simulink model "example_simulink_model_wrapper_firmware"  (R2020b)
settings: Solver=ode2  StartTime=0.0  StopTime=inf  FixedStep=0.01  RelTol=1e-3
undefined symbols (not defined in the file or in its folder): constants
settings Model: Creator=ac112430  LastModifiedBy=ac134326
settings DataIOCC: ReturnWorkspaceOutputs=off
settings OptimizationCC: DefaultParameterBehavior=Inlined  DefaultUnderspecifiedDataType=single  PassReuseOutputArgsAs=Individual arguments  EfficientTunableParamExpr=on
settings DebuggingCC: ParameterPrecisionLossMsg=none  ParameterTunabilityLossMsg=error  ArithmeticOperatorsInVariantConditions=warning
settings HardwareCC: ProdBitPerPointer=32  ProdBitPerSizeT=32  ProdBitPerPtrDiffT=32  ProdLargestAtomicInteger=Long  ProdLargestAtomicFloat=Double  ProdIntDivRoundTo=Undefined  ProdWordSize=32  ProdHWDeviceType=ARM Compatible->ARM Cortex
settings ModelReferenceCC: ModelReferenceNumInstancesAllowed=Single  PropagateSignalLabelsOutOfModel=off
settings SFSimCC: SimUseLocalCustomCode=off  MATLABDynamicMemAlloc=off  CustomCodeUndefinedFunction=UseInterfaceOnly
settings RTWCC: Description=Embedded Coder  SystemTargetFile=ert.tlc  GenCodeOnly=on  TemplateMakefile=ert_default_tmf  RTWUseLocalCustomCode=off  IncludeHyperlinkInReport=on
settings CodeAppCC: IgnoreCustomStorageClasses=off  MaxIdLength=63  StateflowObjectComments=on
settings ERTTargetCC: TargetLangStandard=C99 (ISO)  GenerateSampleERTMain=on  SupportNonFinite=off  SupportComplex=off  InlinedParameterPlacement=NonHierarchical  ERTCustomFileTemplate=example_file_process.tlc  ConvertIfToSwitch=off  SuppressUnreachableDefaultCases=off

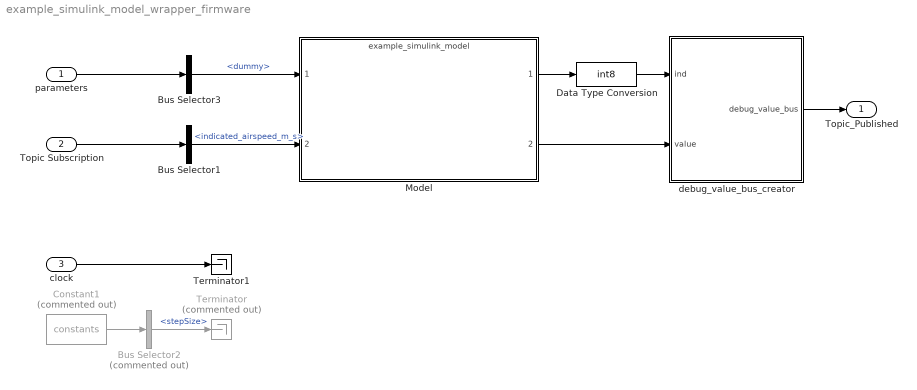
== system example_simulink_model_wrapper_firmware ==
  parameters : Inport  OutDataTypeStr=Bus: parameterBus
  Topic Subscription : Inport  Port=2  OutDataTypeStr=Bus: airspeed_bus
  clock : Inport  Port=3  OutDataTypeStr=single
  Bus Selector1 : BusSelector  OutputSignals=indicated_airspeed_m_s
  Bus Selector2 : BusSelector  Commented=on  OutputSignals=stepSize
  Bus Selector3 : BusSelector  OutputSignals=dummy
  Constant1 : Constant  Commented=on  Value=constants  OutDataTypeStr=Bus: constantsBus
  Data Type Conversion : DataTypeConversion  OutDataTypeStr=int8
  Model : ModelReference  ModelNameDialog=example_simulink_model.slx  SimulationMode=Normal  ModelReferenceVersion=4.3
  Terminator : Terminator  Commented=on
  Terminator1 : Terminator
  debug_value_bus_creator : Subsystem
  Topic_Published : Outport  OutDataTypeStr=Bus: debug_value_bus  SampleTime=[0.01,0]  VectorParamsAs1DForOutWhenUnconnected=off
  wires:
  clock/1 -> Terminator1/1
  parameters/1 -> Bus Selector3/1
  Constant1/1 -> Bus Selector2/1
  Bus Selector2/1 -> Terminator/1  "<stepSize>"
  Topic Subscription/1 -> Bus Selector1/1
  debug_value_bus_creator/1(debug_value_bus) -> Topic_Published/1
  Bus Selector3/1 -> Model/1  "<dummy>"
  Bus Selector1/1 -> Model/2  "<indicated_airspeed_m_s>"
  Model/1 -> Data Type Conversion/1
  Model/2 -> debug_value_bus_creator/2(value)
  Data Type Conversion/1 -> debug_value_bus_creator/1(ind)

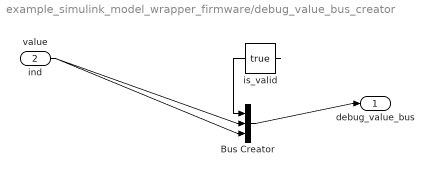
== system example_simulink_model_wrapper_firmware/debug_value_bus_creator ==
  ind : Inport  OutDataTypeStr=int8  PortDimensions=1
  value : Inport  Port=2  OutDataTypeStr=single  PortDimensions=1
  Bus Creator : BusCreator  Inputs=3  OutDataTypeStr=Bus: debug_value_bus
      settings: InheritFromInputs=off
  is_valid : Constant  Value=true  OutDataTypeStr=boolean
  debug_value_bus : Outport  OutDataTypeStr=Bus: debug_value_bus
  wires:
  is_valid/1 -> Bus Creator/1
  ind/1 -> Bus Creator/2
  value/1 -> Bus Creator/3
  Bus Creator/1 -> debug_value_bus/1
